simulink model "dvbs2_stream"  (R2024b)
settings: Solver=FixedStepDiscrete  StartTime=0.0  StopTime=18000/Fs  RelTol=1e-3
PreLoadFcn:
  | Rs = 125e3;
  | Fs = 8*Rs;
  | nsamp = 4096;
  | t = (0:nsamp)/Fs;
  | y = randi(2^8-1,1,2048);
  | ly = length(y);
InitFcn:
  | Rs = 125e3;
  | Fs = 8*Rs;
  | nsamp = 4096;
  | t = (0:nsamp)/Fs;
  | y = randi(2^8-1,1,2048);
  | ly = length(y);
libraries: hdlsllib x132, simulink x41, dspsigops x7, commseqgen3 x5, whdlutilities x5, commhdlcrc x2, dsphdlfiltering2 x1, whdlmod x1, sdrzblksprivate x1
(part 2 of 6)

== system dvbs2_stream/HDL_DUT/Tx/DVB-S2 Tx/BB Frame Generator/Multiplexer ==
  dataBits : Inport
  dataValid : Inport  Port=2
  dataEnd : Inport  Port=3
  headerBits : Inport  Port=4
  headerStart : Inport  Port=5
  headerValid : Inport  Port=6
  MODCOD : Inport  Port=7
  FECFrame : Inport  Port=8
  Delay{,1..3} (4 alike) : Delay
  Delay4 : Delay  DelayLength=1
  Delay5 : Delay  DelayLength=1
  Logical Operator : Logic  Operator=OR  AllPortsSameDT=off  OutDataTypeStr=boolean
  No HDL : Subsystem
  Switch : Switch  Criteria=u2 ~= 0  SaturateOnIntegerOverflow=off  InputSameDT=off
  dataOut : Outport
  startOut : Outport  Port=2
  endOut : Outport  Port=3
  validOut : Outport  Port=4
  MODCODOut : Outport  Port=5
  FECFrameOut : Outport  Port=6
  wires:
  FECFrame/1 -> Delay5/1
  Delay5/1 -> FECFrameOut/1
  Delay4/1 -> MODCODOut/1
  Delay3/1 -> endOut/1
  Delay2/1 -> startOut/1
  Delay1/1 -> validOut/1
  Delay/1 -> dataOut/1
  dataValid/1 -> No HDL/1(dvalid), Logical Operator/1, Switch/2
  MODCOD/1 -> Delay4/1
  Logical Operator/1 -> Delay1/1
  Switch/1 -> Delay/1
  headerValid/1 -> No HDL/2(hvalid), Logical Operator/2
  headerBits/1 -> Switch/3
  dataBits/1 -> Switch/1
  dataEnd/1 -> Delay3/1
  headerStart/1 -> Delay2/1

== system dvbs2_stream/HDL_DUT/Tx/DVB-S2 Tx/FEC Encoder/DVB-S2 BCH Encoder ==
  dataIn : Inport
  ctrlIn : Inport  Port=2
  frameType : Inport  Port=3
  codeRateIdx : Inport  Port=4
  Input controller : Subsystem
  Output Controller : Subsystem
  Parity Generation : Subsystem
  Store and Retreive Input : Subsystem
  Terminator : Terminator
  dataOut : Outport
  ctrlOut : Outport  Port=2
  wires:
  Store and Retreive Input/2(outrd_data) -> Parity Generation/1(outrd_data)
  Store and Retreive Input/3(outRd_valid) -> Parity Generation/2(outRd_valid)
  Output Controller/1(outData) -> dataOut/1
  Output Controller/2(outCtrl) -> ctrlOut/1
  Store and Retreive Input/4(ParityCalCompFlag) -> Parity Generation/3(ParityCalCompFlag)
  Parity Generation/3(parityScalarOut) -> Output Controller/4(outputParity)
  Parity Generation/4(parityScalarValidOut) -> Output Controller/5(validParity)
  Output Controller/3(nxtFrame) -> Terminator/1
  Input controller/6(reset) -> Store and Retreive Input/7(resetIn)
  ctrlIn/1 -> Input controller/1(ctrlIn)
  frameType/1 -> Input controller/2(frameType)
  codeRateIdx/1 -> Input controller/3(codeRateIdx)
  Input controller/1(iwr_enb) -> Store and Retreive Input/2(iwr_enb)
  Input controller/8(sampledStartIn) -> Output Controller/8(sampledStartIn)
  Input controller/2(iwr_addr) -> Store and Retreive Input/3(iwr_addr)
  Input controller/5(framLenDelayed) -> Store and Retreive Input/6(framLenDelayed)
  Input controller/3(ird_addr) -> Store and Retreive Input/4(ird_addr)
  Input controller/7(parLen) -> Output Controller/7(parLen), Parity Generation/5(parLen)
  Input controller/4(ird_valid) -> Store and Retreive Input/5(ird_valid)
  Input controller/11(frameLen) -> Output Controller/11(frameLen)
  Input controller/12(validCodeRate) -> Output Controller/12(validCodeRate)
  Input controller/13(unitFrameLen) -> Output Controller/13(unitFrameLen)
  dataIn/1 -> Store and Retreive Input/1(iwr_data)
  Store and Retreive Input/5(resetOut) -> Parity Generation/4(resetIn)
  Parity Generation/5(resetOut) -> Output Controller/6(resetIn)
  Parity Generation/1(readDataOut) -> Output Controller/2(outputMsg)
  Parity Generation/2(readValidOut) -> Output Controller/3(validMsg)
  Store and Retreive Input/1(framLenDelay) -> Output Controller/1(framLenDelayed)
  Input controller/9(enbBCHEnc) -> Output Controller/9(enbBCHEnc)
  Input controller/10(sampledEndIn) -> Output Controller/10(sampledEndIn)

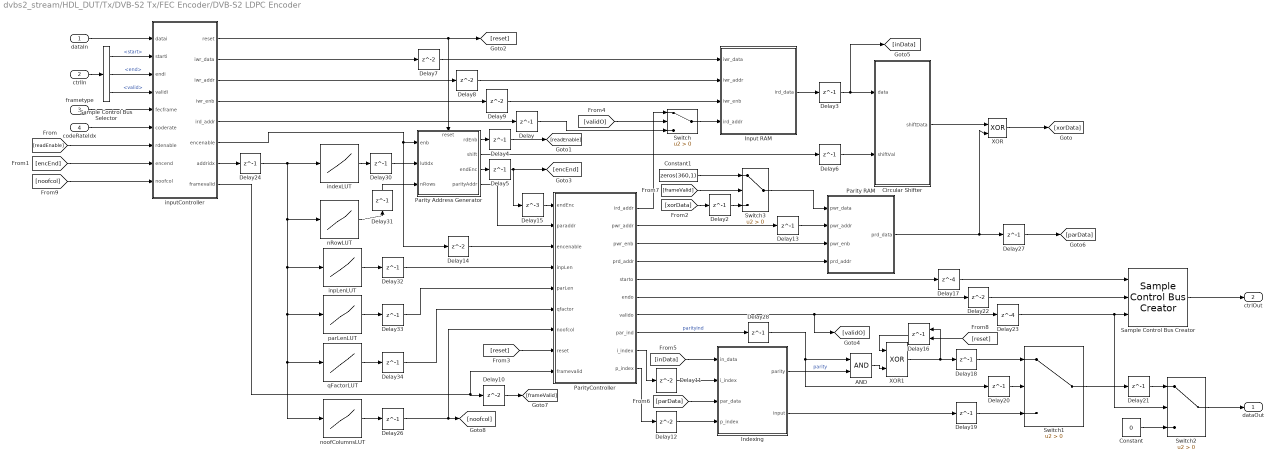
== system dvbs2_stream/HDL_DUT/Tx/DVB-S2 Tx/FEC Encoder/DVB-S2 LDPC Encoder ==
  dataIn : Inport
  ctrlIn : Inport  Port=2
  frametype : Inport  Port=3
  codeRateIdx : Inport  Port=4
  AND : Logic  IconShape=distinctive  AllPortsSameDT=off  OutDataTypeStr=boolean
  Circular Shifter : Subsystem
  Constant : Constant  Value=0  OutDataTypeStr=boolean  SampleTime=-1
  Constant1 : Constant  Value=zeros(360,1)  OutDataTypeStr=boolean  SampleTime=-1
  Delay{,2..6,13,18..21,24,26..28,30..34} (20 alike) : Delay  DelayLength=1
  Delay{7..10,14,22} (6 alike) : Delay
  Delay11 : Delay  InitialCondition=1
  Delay12 : Delay  InitialCondition=1
  Delay15 : Delay  DelayLength=3
  Delay16 : Delay  DelayLength=1  ExternalReset=Level
      settings: InputPortMap=u0,r5
  Delay17 : Delay  DelayLength=4
  Delay23 : Delay  DelayLength=4  InitialCondition=0
  Indexing : MATLAB Function  TreatAsAtomicUnit=on
  Input RAM : Subsystem  TreatAsAtomicUnit=on
  Parity Address Generator : Subsystem
      settings: PortSchema="{\"entries\":[{\"content\":{\"sides\":[{\"content\":{\"connectorIds\":[\"In1\",\"In2\",\"In3\"]},\"type\":\"ConnectorPlacement.EquallySpacedRectSide\",\"uuid\":\"3d7dec72-7252-434a-9e41-e0042beb8f81\"},{\"content\":{\"connectorIds\":[\"Out1\",\"Out2\",\"Out3\",\"Out4\"],\"side\":\"RIGHT\"},\"type\":\"ConnectorPlacement.EquallySpacedRectSide\",\"uuid\":\"b52d290b-db9d-4f8b-b785-ddc131f6f7c7\"},{\"content\":{\"connectorIds\":[\"In4\"],\"side\":\"TOP\"},\"type\":\"ConnectorPlacement.EquallySpacedRectSide\",\"uuid\":\"6c6734b1-a517-4502-8814-67d54e3edf46\"}]},\"type\":\"ConnectorPlacement.EquallySpacedConnector\",\"uuid\":\"7bd65a32-b8b8-4f3b-b937-2885ab80089c\"}],\"packageUris\":[\"http://schema.mathworks.com/mf0/Connector/R2020b\"],\"version\":\"1.0\"}"
  Parity RAM : Subsystem  TreatAsAtomicUnit=on
  ParityController : MATLAB Function  TreatAsAtomicUnit=on
  Sample Control Bus Creator : whdlutilities/Sample Control Bus Creator
  Sample Control Bus Selector : whdlutilities/Sample Control Bus Selector  OutputSignals=start,end,valid
  Switch{,1..3} (4 alike) : Switch  Criteria=u2 > Threshold  SaturateOnIntegerOverflow=off  InputSameDT=off
  XOR : Logic  Operator=XOR  IconShape=distinctive  AllPortsSameDT=off  OutDataTypeStr=boolean
  XOR1 : Logic  Operator=XOR  IconShape=distinctive  AllPortsSameDT=off  OutDataTypeStr=fixdt(0,1,0)
  indexLUT : Lookup_n-D  NumberOfTableDimensions=1  BreakpointsSpecification=Even spacing  BreakpointsForDimension1=[1:20]  BreakpointsForDimension1FirstPoint=0  Table=[0,45,105,177,267,375,495,630,774,924,1084,1246,1246,1246,1246,1246,1246,1255,1270,1288,1308,1335,1365,1398,1433,1470,1510,1510,1510,1510,1510,1510]  InterpMethod=Flat  RemoveProtectionInput=on  InternalRulePriority=Speed  OutDataTypeStr=fixdt(0,11,0)  RndMeth=Simplest
  inpLenLUT : Lookup_n-D  NumberOfTableDimensions=1  BreakpointsSpecification=Even spacing  BreakpointsForDimension1=[1:20]  BreakpointsForDimension1FirstPoint=0  Table=[16200,21600,25920,32400,38880,43200,48600,51840,54000,57600,58320,58320,58320,58320,58320,58320,3240,5400,6480,7200,9720,10800,11880,12600,13320,14400,14400,14400,14400,14400,14400,14400]  InterpMethod=Flat  RemoveProtectionInput=on  InternalRulePriority=Speed  OutDataTypeStr=fixdt(0,16,0)  RndMeth=Simplest
  inputController : MATLAB Function  TreatAsAtomicUnit=on
  nRowLUT : Lookup_n-D  NumberOfTableDimensions=1  BreakpointsSpecification=Even spacing  BreakpointsForDimension1=[1:20]  BreakpointsForDimension1FirstPoint=0  Table=[45,60,72,90,108,120,135,144,150,160,162,162,162,162,162,162,9,15,18,20,27,30,33,35,37,40,40,40,40,40,40,40]  InterpMethod=Flat  RemoveProtectionInput=on  InternalRulePriority=Speed  OutDataTypeStr=fixdt(0,8,0)  RndMeth=Simplest
  noofColumnsLUT : Lookup_n-D  NumberOfTableDimensions=1  BreakpointsSpecification=Even spacing  BreakpointsForDimension1=[1:20]  BreakpointsForDimension1FirstPoint=0  Table=[45,60,72,90,108,120,135,144,150,160,162,162,162,162,162,162,9,15,18,20,27,30,33,35,37,40,40,40,40,40,40,40]  InterpMethod=Flat  RemoveProtectionInput=on  InternalRulePriority=Speed  OutDataTypeStr=uint8  RndMeth=Simplest
  parLenLUT : Lookup_n-D  NumberOfTableDimensions=1  BreakpointsSpecification=Even spacing  BreakpointsForDimension1=[1:20]  BreakpointsForDimension1FirstPoint=0  Table=[48600,43200,38880,32400,25920,21600,16200,12960,10800,7200,6480,6480,6480,6480,6480,6480,12960,10800,9720,9000,6480,5400,4320,3600,2880,1800,1800,1800,1800,1800,1800,1800]  InterpMethod=Flat  RemoveProtectionInput=on  InternalRulePriority=Speed  OutDataTypeStr=fixdt(0,16,0)  RndMeth=Simplest
  qFactorLUT : Lookup_n-D  NumberOfTableDimensions=1  BreakpointsSpecification=Even spacing  BreakpointsForDimension1=[1:20]  BreakpointsForDimension1FirstPoint=0  Table=[135,120,108,90,72,60,45,36,30,20,18,18,18,18,18,18,36,30,27,25,18,15,12,10,8,5,5,5,5,5,5,5]  InterpMethod=Flat  RemoveProtectionInput=on  InternalRulePriority=Speed  OutDataTypeStr=fixdt(0,9,0)  RndMeth=Simplest
  dataOut : Outport
  ctrlOut : Outport  Port=2
  wires:
  ParityController/3(pwr_enb) -> Parity RAM/3(pwr_enb)
  noofColumnsLUT/1 -> Delay26/1
  [frameValid] -> Switch3/2
  Input RAM/1(ird_data) -> Delay3/1
  inputController/2(iwr_data) -> Delay7/1
  [xorData] -> Delay2/1
  Delay10/1 -> [frameValid]
  Constant/1 -> Switch2/3
  [noofcol] -> inputController/9(noofcol)
  inputController/6(encenable) -> Parity Address Generator/1(enb), Delay14/1
  [encEnd] -> inputController/8(encend)
  Indexing/2(input) -> Delay19/1
  Delay23/1 -> Switch2/2, Sample Control Bus Creator/3
  ParityController/4(prd_addr) -> Parity RAM/4(prd_addr)
  [reset] -> ParityController/8(reset)
  Delay17/1 -> Sample Control Bus Creator/1
  Delay21/1 -> Switch2/1
  [parData] -> Indexing/3(par_data)
  Delay26/1 -> [noofcol], ParityController/7(noofcol)
  Switch1/1 -> Delay21/1
  Delay33/1 -> ParityController/5(parLen)
  Delay7/1 -> Input RAM/1(iwr_data)
  frametype/1 -> inputController/5(fecframe)
  Delay32/1 -> ParityController/4(inpLen)
  ParityController/1(ird_addr) -> Switch/1
  Delay24/1 -> indexLUT/1, nRowLUT/1, inpLenLUT/1, parLenLUT/1, qFactorLUT/1, noofColumnsLUT/1
  ParityController/6(endo) -> Delay22/1
  Parity Address Generator/1(rdEnb) -> Delay4/1
  Delay11/1 -> Indexing/2(i_index)
  nRowLUT/1 -> Delay31/1
  inputController/5(ird_addr) -> Delay/1
  Sample Control Bus Selector/2 -> inputController/3(endi)  "<end>"
  ParityController/2(pwr_addr) -> Delay13/1
  Delay9/1 -> Input RAM/3(iwr_enb)
  Delay14/1 -> ParityController/3(encenable)
  inpLenLUT/1 -> Delay32/1
  ParityController/10(p_index) -> Delay12/1
  Delay19/1 -> Switch1/3
  [readEnable] -> inputController/7(rdenable)
  Parity Address Generator/3(endEnc) -> Delay5/1
  Delay30/1 -> Parity Address Generator/2(lutIdx)
  Parity Address Generator/4(parityAddr) -> ParityController/2(paraddr)
  [validO] -> Switch/2
  indexLUT/1 -> Delay30/1
  [inData] -> Indexing/1(in_data)
  Sample Control Bus Selector/1 -> inputController/2(starti)  "<start>"
  Delay28/1 -> AND/1, Delay20/1
  Indexing/1(parity) -> AND/2  "parity"
  Delay3/1 -> Circular Shifter/1(data), [inData]
  ctrlIn/1 -> Sample Control Bus Selector/1
  ParityController/8(par_ind) -> Delay28/1  "parityInd"
  Sample Control Bus Creator/1 -> ctrlOut/1
  Delay31/1 -> Parity Address Generator/3(nRows)
  inputController/1(reset) -> [reset], Parity Address Generator/4(reset)
  Delay16/1 -> XOR1/1
  Delay13/1 -> Parity RAM/2(pwr_addr)
  Switch2/1 -> dataOut/1
  AND/1 -> XOR1/2
  Delay12/1 -> Indexing/4(p_index)
  qFactorLUT/1 -> Delay34/1
  ParityController/5(starto) -> Delay17/1
  Delay/1 -> Switch/3
  Delay22/1 -> Sample Control Bus Creator/2
  XOR1/1 -> Delay18/1, Delay16/1
  Delay5/1 -> Delay15/1, [encEnd]
  Parity RAM/1(prd_data) -> XOR/2, Delay27/1
  ParityController/9(i_index) -> Delay11/1
  codeRateIdx/1 -> inputController/6(coderate)
  Switch3/1 -> Parity RAM/1(pwr_data)
  Delay27/1 -> [parData]
  Delay4/1 -> [readEnable]
  Switch/1 -> Input RAM/4(ird_addr)
  Circular Shifter/1(shiftData) -> XOR/1
  Constant1/1 -> Switch3/1
  dataIn/1 -> inputController/1(datai)
  Delay15/1 -> ParityController/1(endEnc)
  Delay34/1 -> ParityController/6(qfactor)
  Delay2/1 -> Switch3/3
  Delay8/1 -> Input RAM/2(iwr_addr)
  Delay6/1 -> Circular Shifter/2(shiftVal)
  parLenLUT/1 -> Delay33/1
  Delay20/1 -> Switch1/2
  inputController/3(iwr_addr) -> Delay8/1
  inputController/8(framevalid) -> ParityController/9(framevalid), Delay10/1
  Sample Control Bus Selector/3 -> inputController/4(validi)  "<valid>"
  inputController/4(iwr_enb) -> Delay9/1
  inputController/7(addridx) -> Delay24/1
  Delay18/1 -> Switch1/1
  XOR/1 -> [xorData]
  ParityController/7(valido) -> Delay23/1, [validO]
  Parity Address Generator/2(shift) -> Delay6/1
  [reset] -> Delay16/2

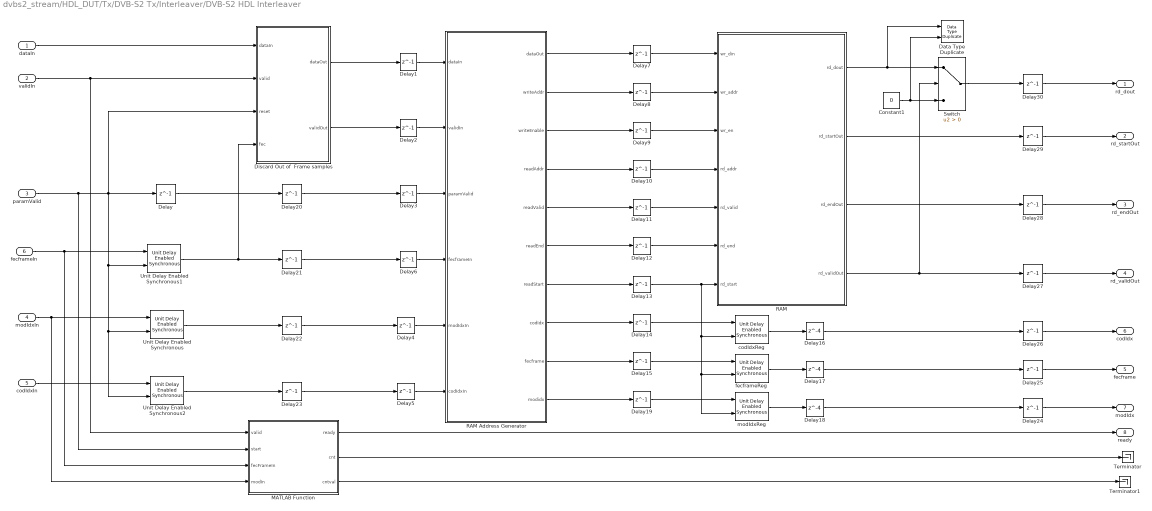
== system dvbs2_stream/HDL_DUT/Tx/DVB-S2 Tx/Interleaver/DVB-S2 HDL Interleaver ==
  dataIn : Inport
  validIn : Inport  Port=2
  paramValid : Inport  Port=3
  modIdxIn : Inport  Port=4
  codIdxIn : Inport  Port=5
  fecframeIn : Inport  Port=6
  Constant1 : Constant  Value=0  OutDataTypeStr=Inherit: Inherit via back propagation  SampleTime=Tsamp
  Data Type Duplicate : DataTypeDuplicate
  Delay{,1..15,19..30} (28 alike) : Delay  DelayLength=1
  Delay16 : Delay  DelayLength=4
  Delay17 : Delay  DelayLength=4
  Delay18 : Delay  DelayLength=4
  Discard Out of  Frame samples : MATLAB Function  TreatAsAtomicUnit=on
  MATLAB Function : MATLAB Function  TreatAsAtomicUnit=on
  RAM : Subsystem
  RAM Address Generator : Subsystem
  Switch : Switch  Criteria=u2 > Threshold  SaturateOnIntegerOverflow=off  InputSameDT=off
  Terminator : Terminator
  Terminator1 : Terminator
  Unit Delay Enabled Synchronous : hdlsllib/Discrete/Unit Delay Enabled Synchronous  InitialCondition=0.0  SampleTime=-1
  Unit Delay Enabled Synchronous1 : hdlsllib/Discrete/Unit Delay Enabled Synchronous  InitialCondition=0.0  SampleTime=-1
  Unit Delay Enabled Synchronous2 : hdlsllib/Discrete/Unit Delay Enabled Synchronous  InitialCondition=0.0  SampleTime=-1
  codIdxReg : hdlsllib/Discrete/Unit Delay Enabled Synchronous  InitialCondition=0.0  SampleTime=-1
  fecframeReg : hdlsllib/Discrete/Unit Delay Enabled Synchronous  InitialCondition=0.0  SampleTime=-1
  modIdxReg : hdlsllib/Discrete/Unit Delay Enabled Synchronous  InitialCondition=0.0  SampleTime=-1
  rd_dout : Outport
  rd_startOut : Outport  Port=2
  rd_endOut : Outport  Port=3
  rd_validOut : Outport  Port=4
  fecframe : Outport  Port=5
  codIdx : Outport  Port=6
  modIdx : Outport  Port=7
  ready : Outport  Port=8
  wires:
  Delay30/1 -> rd_dout/1
  Delay29/1 -> rd_startOut/1
  Delay28/1 -> rd_endOut/1
  Delay27/1 -> rd_validOut/1
  Delay26/1 -> codIdx/1
  Delay25/1 -> fecframe/1
  Delay24/1 -> modIdx/1
  MATLAB Function/3(cntval) -> Terminator1/1
  MATLAB Function/2(cnt) -> Terminator/1
  MATLAB Function/1(ready) -> ready/1
  RAM/2(rd_startOut) -> Delay29/1
  Delay23/1 -> Delay5/1
  Delay22/1 -> Delay4/1
  Delay21/1 -> Delay6/1
  Delay20/1 -> Delay3/1
  Discard Out of  Frame samples/1(dataOut) -> Delay1/1
  Constant1/1 -> Switch/3, Data Type Duplicate/2
  Switch/1 -> Delay30/1
  Discard Out of  Frame samples/2(validOut) -> Delay2/1
  Unit Delay Enabled Synchronous/1 -> Delay22/1
  Unit Delay Enabled Synchronous2/1 -> Delay23/1
  Unit Delay Enabled Synchronous1/1 -> Delay21/1, Discard Out of  Frame samples/4(fec)
  Delay/1 -> Delay20/1
  Delay19/1 -> modIdxReg/1
  RAM Address Generator/10(modidx) -> Delay19/1
  Delay18/1 -> Delay24/1
  modIdxReg/1 -> Delay18/1
  RAM Address Generator/5(readValid) -> Delay11/1
  RAM Address Generator/8(codIdx) -> Delay14/1
  RAM Address Generator/2(writeAddr) -> Delay8/1
  RAM Address Generator/4(readAddr) -> Delay10/1
  RAM Address Generator/7(readStart) -> Delay13/1
  RAM Address Generator/6(readEnd) -> Delay12/1
  RAM Address Generator/9(fecframe) -> Delay15/1
  RAM Address Generator/3(writeEnable) -> Delay9/1
  dataIn/1 -> Discard Out of  Frame samples/1(dataIn)
  RAM Address Generator/1(dataOut) -> Delay7/1
  validIn/1 -> Discard Out of  Frame samples/2(valid), MATLAB Function/1(valid)
  RAM/4(rd_validOut) -> Delay27/1, Switch/2
  paramValid/1 -> MATLAB Function/2(start), Unit Delay Enabled Synchronous1/2, Unit Delay Enabled Synchronous/2, Unit Delay Enabled Synchronous2/2, Delay/1, Discard Out of  Frame samples/3(reset)
  codIdxIn/1 -> Unit Delay Enabled Synchronous2/1
  modIdxIn/1 -> MATLAB Function/4(modIn), Unit Delay Enabled Synchronous/1
  fecframeIn/1 -> MATLAB Function/3(fecFrameIn), Unit Delay Enabled Synchronous1/1
  RAM/3(rd_endOut) -> Delay28/1
  fecframeReg/1 -> Delay17/1
  RAM/1(rd_dout) -> Switch/1, Data Type Duplicate/1
  codIdxReg/1 -> Delay16/1
  Delay1/1 -> RAM Address Generator/1(dataIn)
  Delay2/1 -> RAM Address Generator/2(validIn)
  Delay3/1 -> RAM Address Generator/3(paramValid)
  Delay4/1 -> RAM Address Generator/5(modIdxIn)
  Delay5/1 -> RAM Address Generator/6(codIdxIn)
  Delay6/1 -> RAM Address Generator/4(fecframeIn)
  Delay7/1 -> RAM/1(wr_din)
  Delay8/1 -> RAM/2(wr_addr)
  Delay9/1 -> RAM/3(wr_en)
  Delay10/1 -> RAM/4(rd_addr)
  Delay11/1 -> RAM/5(rd_valid)
  Delay12/1 -> RAM/6(rd_end)
  Delay13/1 -> RAM/7(rd_start), fecframeReg/2, modIdxReg/2, codIdxReg/2
  Delay14/1 -> codIdxReg/1
  Delay15/1 -> fecframeReg/1
  Delay16/1 -> Delay26/1
  Delay17/1 -> Delay25/1

== system dvbs2_stream/HDL_DUT/Tx/DVB-S2 Tx/No HDL/Subsystem ==
  In1 : Inport
  Enable : EnablePort
  To Workspace : ToWorkspace  VariableName=simDummyFrameNos  SaveFormat=Timeseries  SampleTime=-1
      settings: Save2DSignal=2-D array (concatenate along first dimension)
  wires:
  In1/1 -> To Workspace/1

== system dvbs2_stream/HDL_DUT/Tx/DVB-S2 Tx/PL Frame Generator/Frame Length ==
  fecframe : Inport
  modIdx : Inport  Port=2
  Delay2 : Delay  DelayLength=1
  Delay3 : Delay  DelayLength=8
  Normal Frame xFECFrame Length : Lookup_n-D  NumberOfTableDimensions=1  BreakpointsSpecification=Even spacing  BreakpointsForDimension1=[-5:5]  BreakpointsForDimension1FirstPoint=0  Table=64800./log2([4 8 16 32])  TableDataTypeStr=fixdt(0,15,0)  InterpMethod=Flat  InternalRulePriority=Speed  OutDataTypeStr=fixdt(0,15,0)  RndMeth=Simplest
  Short Frame xFECFrame Length : Lookup_n-D  NumberOfTableDimensions=1  BreakpointsSpecification=Even spacing  BreakpointsForDimension1=[-5:5]  BreakpointsForDimension1FirstPoint=0  Table=16200./log2([4 8 16 32])  TableDataTypeStr=fixdt(0,15,0)  InterpMethod=Flat  InternalRulePriority=Speed  OutDataTypeStr=fixdt(0,15,0)  RndMeth=Simplest
  Switch : Switch  Criteria=u2 ~= 0  SaturateOnIntegerOverflow=off  InputSameDT=off
  xFECFrameLength : Outport
  wires:
  Delay3/1 -> Delay2/1
  Delay2/1 -> xFECFrameLength/1
  modIdx/1 -> Normal Frame xFECFrame Length/1, Short Frame xFECFrame Length/1
  fecframe/1 -> Switch/2
  Normal Frame xFECFrame Length/1 -> Switch/3
  Short Frame xFECFrame Length/1 -> Switch/1
  Switch/1 -> Delay3/1

== system dvbs2_stream/HDL_DUT/Tx/DVB-S2 Tx/PL Frame Generator/Multiplexer ==
  plheaderData : Inport
  plheaderStart : Inport  Port=2
  plheaderEnd : Inport  Port=3
  plheaderValid : Inport  Port=4
  pilotdata : Inport  Port=5
  pilotEnd : Inport  Port=6
  pilotValid : Inport  Port=7
  slotsData : Inport  Port=8
  data16SlotsEnd : Inport  Port=9
  slotsValid : Inport  Port=10
  dummyData : Inport  Port=11
  dummyValid : Inport  Port=12
  dummyHeaderSrt : Inport  Port=13
  dummyHeaderEnd : Inport  Port=14
  Logical Operator : Logic  Operator=OR  AllPortsSameDT=off  OutDataTypeStr=boolean
  Logical Operator2 : Logic  Operator=OR  Inputs=4  AllPortsSameDT=off  OutDataTypeStr=boolean
  Logical Operator3 : Logic  Operator=OR  AllPortsSameDT=off  OutDataTypeStr=boolean
  Multiport Switch : MultiPortSwitch  DataPortOrder=Zero-based contiguous  Inputs=4  zeroidx=on  SaturateOnIntegerOverflow=off  InputSameDT=off
  No HDL : Subsystem
  Priority Encoder : MATLAB Function  TreatAsAtomicUnit=on
  Terminator : Terminator
  Terminator11 : Terminator
  dataOut : Outport
  startOfPlheader : Outport  Port=2
  endOfPlheader : Outport  Port=3
  validOut : Outport  Port=4
  wires:
  Logical Operator3/1 -> endOfPlheader/1
  Logical Operator/1 -> startOfPlheader/1
  dummyHeaderEnd/1 -> Logical Operator3/1
  dummyHeaderSrt/1 -> Logical Operator/1
  dummyData/1 -> Multiport Switch/5
  slotsData/1 -> Multiport Switch/4
  pilotdata/1 -> Multiport Switch/3
  plheaderData/1 -> Multiport Switch/2
  plheaderEnd/1 -> Logical Operator3/2
  Multiport Switch/1 -> dataOut/1
  Priority Encoder/1(y) -> Multiport Switch/1
  dummyValid/1 -> Priority Encoder/4(x4), Logical Operator2/4, No HDL/4(dummyValid)
  plheaderStart/1 -> Logical Operator/2
  Logical Operator2/1 -> validOut/1
  pilotEnd/1 -> Terminator11/1
  plheaderValid/1 -> No HDL/2(In2), Logical Operator2/2, Priority Encoder/1(x1)
  data16SlotsEnd/1 -> Terminator/1
  pilotValid/1 -> No HDL/1(In1), Logical Operator2/1, Priority Encoder/2(x2)
  slotsValid/1 -> Logical Operator2/3, No HDL/3(In5), Priority Encoder/3(x3)

== system dvbs2_stream/HDL_DUT/Tx/DVB-S2 Tx/PL Frame Generator/PL Data Scrambler ==
  dataIn : Inport
  startOfPlheader : Inport  Port=2
  endOfPlheader : Inport  Port=3
  validIn : Inport  Port=4
  Delay1 : Delay  DelayLength=7
  Delay{2..8,10..12,22..26} (15 alike) : Delay  DelayLength=1
  Delay{13..21} (9 alike) : Delay
  Delay9 : Delay  DelayLength=7
  PL Scramble Sequence Mapper LUT : Lookup_n-D  NumberOfTableDimensions=1  LookupTableObject=''  BreakpointsSpecification=Even spacing  BreakpointsForDimension1=[-5:5]  BreakpointsForDimension1FirstPoint=0  BreakpointsForDimension2FirstPoint=10  BreakpointsForDimension2Spacing=12  IndexSearchMethod=Evenly spaced points  Table=[1;1i;-1;-1i]  TableDataTypeStr=fixdt(1,2,0)  InterpMethod=Flat  DiagnosticForOutOfRangeInput=Error  InternalRulePriority=Speed  OutDataTypeStr=fixdt(1,2,0)  RndMeth=Simplest
  PL Scrambler Gold Sequence Generator : Subsystem  mask{n=0}
      mask prompts: n "Index of Gold Sequence :"
  Product : Product  OutDataTypeStr=Inherit: Same as first input
  Switch : Switch  Criteria=u2 ~= 0  SaturateOnIntegerOverflow=off  InputSameDT=off
  Unit Delay Enabled Resettable Synchronous : hdlsllib/Discrete/Unit Delay Enabled Resettable Synchronous  InitialCondition=0.0  SampleTime=-1
  dataOut : Outport
  validOut : Outport  Port=2
  wires:
  Unit Delay Enabled Resettable Synchronous/1 -> Delay1/1
  Delay26/1 -> PL Scrambler Gold Sequence Generator/1(reset), Unit Delay Enabled Resettable Synchronous/3
  Delay25/1 -> PL Scrambler Gold Sequence Generator/2(validIn)
  Delay24/1 -> Delay9/1
  startOfPlheader/1 -> Unit Delay Enabled Resettable Synchronous/1, Unit Delay Enabled Resettable Synchronous/2
  PL Scrambler Gold Sequence Generator/1(dataOut) -> Delay2/1
  Delay11/1 -> Delay14/1
  Delay7/1 -> Delay16/1
  dataIn/1 -> Delay24/1
  PL Scramble Sequence Mapper LUT/1 -> Delay7/1
  Product/1 -> Delay20/1
  Switch/1 -> Delay22/1
  PL Scrambler Gold Sequence Generator/2(validOut) -> Delay5/1
  endOfPlheader/1 -> Delay26/1
  validIn/1 -> Delay25/1
  Delay9/1 -> Delay4/1, Delay6/1
  Delay1/1 -> Delay3/1
  Delay2/1 -> PL Scramble Sequence Mapper LUT/1
  Delay3/1 -> Delay11/1
  Delay4/1 -> Delay10/1
  Delay5/1 -> Delay8/1
  Delay6/1 -> Delay12/1
  Delay8/1 -> Delay17/1
  Delay10/1 -> Delay15/1
  Delay13/1 -> Delay18/1
  Delay14/1 -> Delay19/1
  Delay15/1 -> Product/1
  Delay16/1 -> Product/2
  Delay17/1 -> Delay21/1
  Delay18/1 -> Switch/1
  Delay19/1 -> Switch/2
  Delay20/1 -> Switch/3
  Delay21/1 -> Delay23/1
  Delay22/1 -> dataOut/1
  Delay23/1 -> validOut/1
  Delay12/1 -> Delay13/1

== system dvbs2_stream/HDL_DUT/Tx/DVB-S2 Tx/PL Frame Generator/PL Header Generator ==
  trigger : Inport
  pilotActive : Inport  Port=2
  modcod : Inport  Port=3
  fecframe : Inport  Port=4
  Delay{,1..3} (4 alike) : Delay  DelayLength=1
  PL Header Bits Generator : Subsystem
  Terminator : Terminator
  Terminator1 : Terminator
  piby2 BPSK Modulator : Subsystem
  dataOut : Outport
  validOut : Outport  Port=2
  wires:
  piby2 BPSK Modulator/2(startOut) -> Terminator/1
  piby2 BPSK Modulator/1(dataOut) -> dataOut/1
  piby2 BPSK Modulator/3(endOut) -> Terminator1/1
  PL Header Bits Generator/3(bitsEnd) -> piby2 BPSK Modulator/3(endIn)
  PL Header Bits Generator/2(bitsStart) -> piby2 BPSK Modulator/2(startIn)
  piby2 BPSK Modulator/4(validOut) -> validOut/1
  PL Header Bits Generator/4(bitsValid) -> piby2 BPSK Modulator/4(validIn)
  PL Header Bits Generator/1(bitsOut) -> piby2 BPSK Modulator/1(bitsIn)
  Delay3/1 -> PL Header Bits Generator/1(trigger)
  Delay2/1 -> PL Header Bits Generator/2(pilotActive)
  Delay1/1 -> PL Header Bits Generator/3(modcod)
  Delay/1 -> PL Header Bits Generator/4(fecframe)
  pilotActive/1 -> Delay2/1
  modcod/1 -> Delay1/1
  fecframe/1 -> Delay/1
  trigger/1 -> Delay3/1

== system dvbs2_stream/HDL_DUT/Tx/DVB-S2 Tx/PL Frame Generator/RAM FIFO ==
  dataIn : Inport
  validIn : Inport  Port=2
  dataIn1 : Inport  Port=3
  startIn1 : Inport  Port=4
  validIn1 : Inport  Port=5
  frameLength : Inport  Port=6
  PL Data FIFO : Subsystem
      settings: PortSchema="{\"entries\":[{\"content\":{\"sides\":[{\"content\":{\"connectorIds\":[\"In1\",\"In2\",\"Out8\",\"In3\",\"In4\",\"In5\",\"In6\"]},\"type\":\"ConnectorPlacement.EquallySpacedRectSide\",\"uuid\":\"8624b1c3-ba7c-4e35-b094-1d3a75bbb5aa\"},{\"content\":{\"connectorIds\":[\"Out1\",\"Out2\",\"Out3\",\"Out4\",\"Out5\",\"Out6\",\"Out7\"],\"side\":\"RIGHT\"},\"type\":\"ConnectorPlacement.EquallySpacedRectSide\",\"uuid\":\"28b8a943-c986-4665-8db5-1a3b0585df3a\"},{\"content\":{\"connectorIds\":[],\"side\":\"TOP\"},\"type\":\"ConnectorPlacement.EquallySpacedRectSide\",\"uuid\":\"814d6e08-8c72-454b-9b48-c3c62ce2dfb2\"}]},\"type\":\"ConnectorPlacement.EquallySpacedConnector\",\"uuid\":\"82423169-df73-4f70-a83d-ba96081f6481\"}],\"packageUris\":[\"http://schema.mathworks.com/mf0/Connector/R2020b\"],\"version\":\"1.0\"}"
  PL Header FIFO : Subsystem
      settings: PortSchema="{\"entries\":[{\"content\":{\"sides\":[{\"content\":{\"connectorIds\":[\"In1\",\"In2\",\"In3\",\"Out5\"]},\"type\":\"ConnectorPlacement.EquallySpacedRectSide\",\"uuid\":\"17ee1903-61f4-462b-918b-37a4577cd6d5\"},{\"content\":{\"connectorIds\":[\"Out1\",\"Out2\",\"Out3\",\"Out4\"],\"side\":\"RIGHT\"},\"type\":\"ConnectorPlacement.EquallySpacedRectSide\",\"uuid\":\"53e99393-0da1-48e4-bd02-4cd54a66bf15\"},{\"content\":{\"connectorIds\":[],\"side\":\"TOP\"},\"type\":\"ConnectorPlacement.EquallySpacedRectSide\",\"uuid\":\"3f5b7744-cb83-4728-90ec-96c952f929fa\"}]},\"type\":\"ConnectorPlacement.EquallySpacedConnector\",\"uuid\":\"7c0ee041-1408-4d92-8895-be25a9dc4cb3\"}],\"packageUris\":[\"http://schema.mathworks.com/mf0/Connector/R2020b\"],\"version\":\"1.0\"}"
  Pilot Generator : Subsystem
      settings: PortSchema="{\"entries\":[{\"content\":{\"sides\":[{\"content\":{\"connectorIds\":[\"Out4\"]},\"type\":\"ConnectorPlacement.EquallySpacedRectSide\",\"uuid\":\"60393444-e96f-4a49-aa63-e73913838962\"},{\"content\":{\"connectorIds\":[\"Out1\",\"Out2\",\"Out3\",\"In1\"],\"side\":\"RIGHT\"},\"type\":\"ConnectorPlacement.EquallySpacedRectSide\",\"uuid\":\"bbfeed4a-cbdf-4f6b-9c28-37958929d3d3\"},{\"content\":{\"connectorIds\":[],\"side\":\"TOP\"},\"type\":\"ConnectorPlacement.EquallySpacedRectSide\",\"uuid\":\"3a1e215d-56d0-454b-a618-c727de9dda1a\"}]},\"type\":\"ConnectorPlacement.EquallySpacedConnector\",\"uuid\":\"0bef8ac2-da74-4396-b0bf-efe44cab5a13\"}],\"packageUris\":[\"http://schema.mathworks.com/mf0/Connector/R2020b\"],\"version\":\"1.0\"}"
  plheaderData : Outport
  plheaderStart : Outport  Port=2
  plheaderEnd : Outport  Port=3
  plheaderValid : Outport  Port=4
  pilotData : Outport  Port=5
  pilotEnd : Outport  Port=6
  pilotValid : Outport  Port=7
  slotsData : Outport  Port=8
  data16SlotsEnd : Outport  Port=9
  slotsValid : Outport  Port=10
  dummyData : Outport  Port=11
  dummyValid : Outport  Port=12
  dummyHeaderSrt : Outport  Port=13
  dummyHeaderEnd : Outport  Port=14
  wires:
  PL Data FIFO/7(dummyHeaderEnd) -> dummyHeaderEnd/1
  PL Data FIFO/6(dummyHeaderSrt) -> dummyHeaderSrt/1
  PL Data FIFO/5(dummyValid) -> dummyValid/1
  PL Data FIFO/4(dummyData) -> dummyData/1
  startIn1/1 -> PL Data FIFO/4(startIn)
  PL Header FIFO/5(endOut1) -> PL Data FIFO/2(endOfPLHeader)
  Pilot Generator/3(validOut) -> pilotValid/1
  PL Header FIFO/2(startOut) -> plheaderStart/1
  PL Data FIFO/2(dataOut) -> slotsData/1
  Pilot Generator/1(dataOut) -> pilotData/1
  frameLength/1 -> PL Data FIFO/6(frameLength)
  validIn1/1 -> PL Data FIFO/5(validIn)
  PL Data FIFO/3(validOut) -> slotsValid/1
  dataIn1/1 -> PL Data FIFO/3(dataIn)
  PL Header FIFO/1(dataOut) -> plheaderData/1
  validIn/1 -> PL Header FIFO/2(validIn)
  Pilot Generator/2(endOut) -> pilotEnd/1
  PL Header FIFO/3(endOut) -> plheaderEnd/1
  PL Header FIFO/4(validOut) -> plheaderValid/1
  dataIn/1 -> PL Header FIFO/1(dataIn)
  PL Data FIFO/1(endOf16Slots) -> Pilot Generator/1(trigger), data16SlotsEnd/1
  Pilot Generator/4(endOut1) -> PL Data FIFO/1(endOfPilotBlk)
  PL Data FIFO/8(nextFrameReady) -> PL Header FIFO/3(nextFrameReady)

== system dvbs2_stream/HDL_DUT/Tx/DVB-S2 Tx/PL Frame Generator/Subsystem ==
  data : Inport
  start : Inport  Port=2
  endIn : Inport  Port=3
  validIn : Inport  Port=4
  8x : MATLAB Function  TreatAsAtomicUnit=on
  Delay : Delay  DelayLength=8
  Delay1 : Delay  DelayLength=8
  Delay2 : Delay  DelayLength=1
  Unit Delay Enabled Synchronous : hdlsllib/Discrete/Unit Delay Enabled Synchronous  InitialCondition=0.0  SampleTime=-1
  dataOut : Outport
  startOut : Outport  Port=2
  validOut : Outport  Port=3
  wires:
  Delay2/1 -> dataOut/1
  Unit Delay Enabled Synchronous/1 -> Delay2/1
  Delay1/1 -> 8x/2(endIn)
  Delay/1 -> 8x/1(startIn)
  endIn/1 -> Delay1/1
  start/1 -> Delay/1
  validIn/1 -> Unit Delay Enabled Synchronous/2
  data/1 -> Unit Delay Enabled Synchronous/1
  8x/1(startOut) -> startOut/1
  8x/2(validOut) -> validOut/1

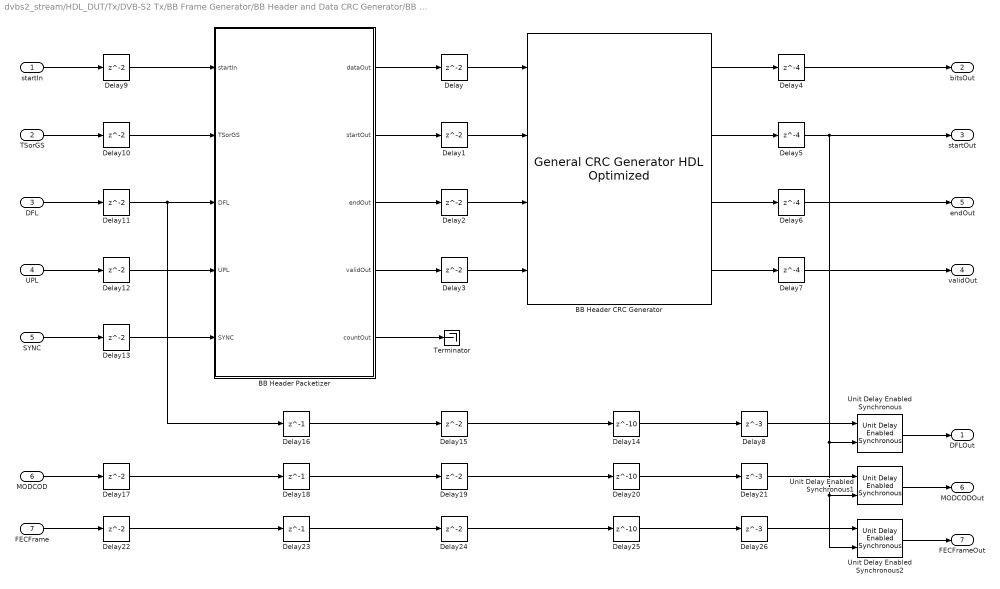
== system dvbs2_stream/HDL_DUT/Tx/DVB-S2 Tx/BB Frame Generator/BB Header and Data CRC Generator/BB Header Generator ==
  startIn : Inport
  TSorGS : Inport  Port=2
  DFL : Inport  Port=3
  UPL : Inport  Port=4
  SYNC : Inport  Port=5
  MODCOD : Inport  Port=6
  FECFrame : Inport  Port=7
  BB Header CRC Generator : commhdlcrc/General CRC Generator HDL Optimized  Polynomial=[1 1 1 0 1 0 1 0 1]  InitialState=0  DirectMethod=off  ReflectInput=off  ReflectCRCChecksum=off  FinalXORValue=0  SimulateUsing=Code generation
  BB Header Packetizer : MATLAB Function  TreatAsAtomicUnit=on
  Delay{,1..3,9..13,15,17,19,22,24} (14 alike) : Delay
  Delay14 : Delay  DelayLength=10
  Delay16 : Delay  DelayLength=1
  Delay18 : Delay  DelayLength=1
  Delay20 : Delay  DelayLength=10
  Delay21 : Delay  DelayLength=3
  Delay23 : Delay  DelayLength=1
  Delay25 : Delay  DelayLength=10
  Delay26 : Delay  DelayLength=3
  Delay{4..7} (4 alike) : Delay  DelayLength=4
  Delay8 : Delay  DelayLength=3
  Terminator : Terminator
  Unit Delay Enabled Synchronous : hdlsllib/Discrete/Unit Delay Enabled Synchronous  InitialCondition=0.0  SampleTime=-1
  Unit Delay Enabled Synchronous1 : hdlsllib/Discrete/Unit Delay Enabled Synchronous  InitialCondition=0.0  SampleTime=-1
  Unit Delay Enabled Synchronous2 : hdlsllib/Discrete/Unit Delay Enabled Synchronous  InitialCondition=0.0  SampleTime=-1
  DFLOut : Outport
  bitsOut : Outport  Port=2
  startOut : Outport  Port=3
  validOut : Outport  Port=4
  endOut : Outport  Port=5
  MODCODOut : Outport  Port=6
  FECFrameOut : Outport  Port=7
  wires:
  Delay26/1 -> Unit Delay Enabled Synchronous2/1
  Delay25/1 -> Delay26/1
  Delay24/1 -> Delay25/1
  Delay23/1 -> Delay24/1
  Delay22/1 -> Delay23/1
  Unit Delay Enabled Synchronous2/1 -> FECFrameOut/1
  FECFrame/1 -> Delay22/1
  Unit Delay Enabled Synchronous1/1 -> MODCODOut/1
  Delay21/1 -> Unit Delay Enabled Synchronous1/1
  Delay20/1 -> Delay21/1
  Delay19/1 -> Delay20/1
  Delay18/1 -> Delay19/1
  Delay17/1 -> Delay18/1
  MODCOD/1 -> Delay17/1
  Delay5/1 -> Unit Delay Enabled Synchronous/2, Unit Delay Enabled Synchronous1/2, Unit Delay Enabled Synchronous2/2, startOut/1
  Unit Delay Enabled Synchronous/1 -> DFLOut/1
  Delay16/1 -> Delay15/1
  Delay11/1 -> Delay16/1, BB Header Packetizer/3(DFL)
  Delay15/1 -> Delay14/1
  Delay14/1 -> Delay8/1
  Delay8/1 -> Unit Delay Enabled Synchronous/1
  Delay13/1 -> BB Header Packetizer/5(SYNC)
  Delay12/1 -> BB Header Packetizer/4(UPL)
  Delay10/1 -> BB Header Packetizer/2(TSorGS)
  Delay9/1 -> BB Header Packetizer/1(startIn)
  Delay7/1 -> validOut/1
  Delay6/1 -> endOut/1
  Delay4/1 -> bitsOut/1
  Delay3/1 -> BB Header CRC Generator/4
  Delay2/1 -> BB Header CRC Generator/3
  Delay1/1 -> BB Header CRC Generator/2
  Delay/1 -> BB Header CRC Generator/1
  BB Header Packetizer/5(countOut) -> Terminator/1
  BB Header CRC Generator/3 -> Delay6/1
  BB Header CRC Generator/4 -> Delay7/1
  BB Header CRC Generator/2 -> Delay5/1
  UPL/1 -> Delay12/1
  BB Header CRC Generator/1 -> Delay4/1
  BB Header Packetizer/1(dataOut) -> Delay/1
  startIn/1 -> Delay9/1
  DFL/1 -> Delay11/1
  BB Header Packetizer/4(validOut) -> Delay3/1
  BB Header Packetizer/2(startOut) -> Delay1/1
  BB Header Packetizer/3(endOut) -> Delay2/1
  SYNC/1 -> Delay13/1
  TSorGS/1 -> Delay10/1

== system dvbs2_stream/HDL_DUT/Tx/DVB-S2 Tx/BB Frame Generator/BB Header and Data CRC Generator/Data Field Generator ==
  dataIn : Inport
  startIn : Inport  Port=2
  endIn : Inport  Port=3
  validIn : Inport  Port=4
  frameEnd : Inport  Port=5
  frameStart : Inport  Port=6
  UPL : Inport  Port=7
  Compare To Constant : simulink/Logic and Bit Operations/Compare To Constant  relop=~=  const=0  OutDataTypeStr=boolean
  Continuous Streams : Subsystem
  Packetized Streams : Subsystem
  Switch{,1..3} (4 alike) : Switch  Criteria=u2 ~= 0  SaturateOnIntegerOverflow=off  InputSameDT=off
  pktBits : Outport
  pktValid : Outport  Port=2
  frameStartOut : Outport  Port=3
  frameEndOut : Outport  Port=4
  wires:
  Compare To Constant/1 -> Switch/2, Switch1/2, Switch2/2, Switch3/2
  UPL/1 -> Compare To Constant/1
  frameStart/1 -> Packetized Streams/6(frameStart), Continuous Streams/4(frameStart)
  frameEnd/1 -> Packetized Streams/5(frameEnd), Continuous Streams/3(frameEnd)
  Continuous Streams/1(dataOut) -> Switch/3
  Continuous Streams/2(validOut) -> Switch1/3
  Continuous Streams/4(frameStartOut) -> Switch3/3
  Continuous Streams/3(frameEndOut) -> Switch2/3
  Switch3/1 -> frameStartOut/1
  Switch2/1 -> frameEndOut/1
  Switch1/1 -> pktValid/1
  Switch/1 -> pktBits/1
  Packetized Streams/4(frameStartOut) -> Switch3/1
  Packetized Streams/3(frameEndOut) -> Switch2/1
  Packetized Streams/2(pktValid) -> Switch1/1
  Packetized Streams/1(pktBits) -> Switch/1
  validIn/1 -> Packetized Streams/4(validIn), Continuous Streams/2(validIn)
  endIn/1 -> Packetized Streams/3(endIn)
  startIn/1 -> Packetized Streams/2(startIn)
  dataIn/1 -> Packetized Streams/1(dataIn), Continuous Streams/1(dataIn)

== system dvbs2_stream/HDL_DUT/Tx/DVB-S2 Tx/BB Frame Generator/BB Header and Data CRC Generator/No HDL ==
  In2 : Inport
  u : Inport  Port=2
  vld : Inport  Port=3
  Logical Operator3 : Logic  Operator=NOT  AllPortsSameDT=off  OutDataTypeStr=boolean
  Logical Operator4 : Logic  AllPortsSameDT=off  OutDataTypeStr=boolean
  Logical Operator5 : Logic  Operator=NOT  AllPortsSameDT=off  OutDataTypeStr=boolean
  MATLAB Function1 : MATLAB Function  TreatAsAtomicUnit=on
  No HDL : Subsystem
  wires:
  Logical Operator3/1 -> Logical Operator4/1
  MATLAB Function1/1(y) -> Logical Operator5/1
  u/1 -> MATLAB Function1/1(u)
  vld/1 -> No HDL/2(vld)
  Logical Operator5/1 -> Logical Operator4/2
  Logical Operator4/1 -> No HDL/1(rdy)
  In2/1 -> Logical Operator3/1

== system dvbs2_stream/HDL_DUT/Tx/DVB-S2 Tx/BB Frame Generator/BB Scrambler/Subsystem ==
  In1 : Inport
  Enable : EnablePort
  PN Sequence Generator : commseqgen3/PN Sequence Generator  poly='z^15 + z + 1'  ini_sta=[1 0 0 1 0 1 0 1 0 0 0 0 0 0 0]  outBitMaskSource=Dialog parameter  shift=15  outVarSiz=off  maxOutSizeMode=Dialog parameter  maxOutSize=[10 1]  Ts=-1  sampPerFrame=1  reset=on  bitPackedOutputs=off  outDataType=Smallest unsigned integer  numPackedBits=8  bitPackDataSigned=off  bitPackedOutDType=double
  Out1 : Outport  InitialOutput=0
  wires:
  PN Sequence Generator/1 -> Out1/1
  In1/1 -> PN Sequence Generator/1

== system dvbs2_stream/HDL_DUT/Tx/DVB-S2 Tx/BB Frame Generator/Data Store FIFO/No HDL ==
  rd : Inport
  wr : Inport  Port=2
  No HDL : Subsystem
  RAM status : MATLAB Function  TreatAsAtomicUnit=on
  wires:
  RAM status/2(ncount) -> No HDL/3(ncount)
  RAM status/3(empty) -> No HDL/4(empty)
  RAM status/1(full) -> No HDL/2(full)
  wr/1 -> RAM status/1(wr), No HDL/1(wr)
  rd/1 -> RAM status/2(rd), No HDL/5(rd)

== system dvbs2_stream/HDL_DUT/Tx/DVB-S2 Tx/BB Frame Generator/Multiplexer/No HDL ==
  dvalid : Inport
  hvalid : Inport  Port=2
  Assertion : Assertion
  Delay : Delay  DelayLength=10
  Logical Operator1 : Logic  AllPortsSameDT=off  OutDataTypeStr=boolean
  Logical Operator2 : Logic  Operator=NOT  AllPortsSameDT=off  OutDataTypeStr=boolean
  wires:
  Delay/1 -> Logical Operator2/1
  dvalid/1 -> Logical Operator1/1
  Logical Operator1/1 -> Delay/1
  hvalid/1 -> Logical Operator1/2
  Logical Operator2/1 -> Assertion/1

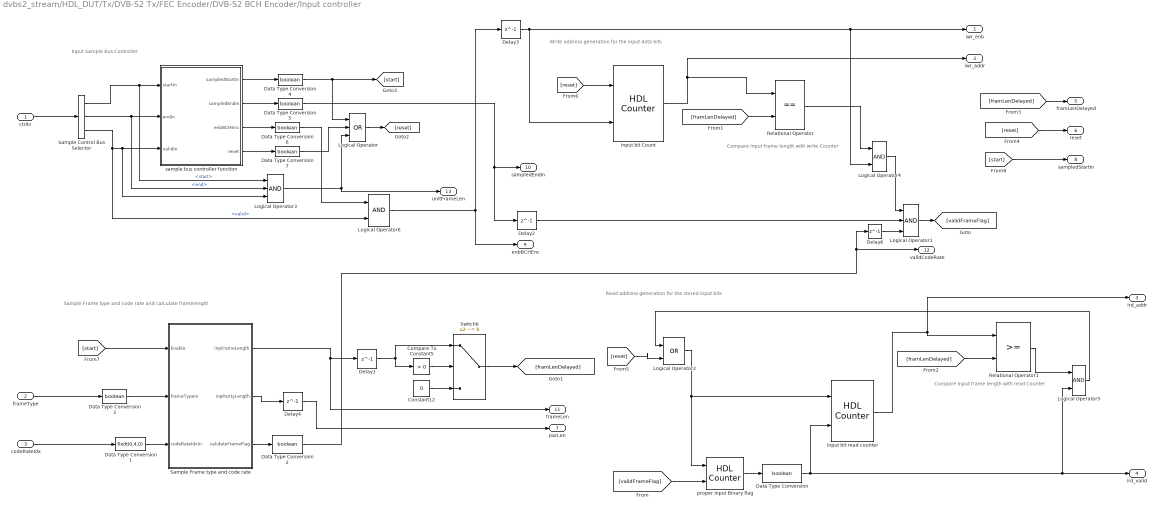
== system dvbs2_stream/HDL_DUT/Tx/DVB-S2 Tx/FEC Encoder/DVB-S2 BCH Encoder/Input controller ==
  note: Input Sample Bus Controller
  note: Compare input frame length with read Counter
  note: Compare input frame length with write Counter
  note: Sample Frame type and code rate and calculate framelength
  note: Write address generation for the input data bits
  note: Read address generation for the stored input bits
  ctrlIn : Inport
  frameType : Inport  Port=2
  codeRateIdx : Inport  Port=3
  Compare To Constant5 : simulink/Logic and Bit Operations/Compare To Constant  relop=>  const=0  OutDataTypeStr=boolean
  Constant12 : Constant  Value=0  OutDataTypeStr=Inherit: Inherit via back propagation  SampleTime=-1
  Data Type Conversion{,2,4..7} (6 alike) : DataTypeConversion  OutDataTypeStr=boolean  SaturateOnIntegerOverflow=off  RndMeth=Floor
  Data Type Conversion1 : DataTypeConversion  OutDataTypeStr=fixdt(0,4,0)  RndMeth=Nearest  SaturateOnIntegerOverflow=off
  Data Type Conversion3 : DataTypeConversion  OutDataTypeStr=boolean  RndMeth=Nearest  SaturateOnIntegerOverflow=off
  Delay{1..4,6} (5 alike) : Delay  DelayLength=1
  Input bit Count : hdlsllib/Sources/HDL Counter  CountType=Count limited  CountInit=0  CountStep=1  CountMax=65535  CountFromType=Initial value  CountFrom=0  CountResetPort=on  CountLoadPort=off  CountEnbPort=on  CountDirPort=off  CountHitOutputPort=off  CountDataType=Unsigned  CountWordLen=16  CountFracLen=0  CountSampTime=1
  Logical Operator : Logic  Operator=OR  Inputs=3  IconShape=distinctive  AllPortsSameDT=off  OutDataTypeStr=boolean
  Logical Operator1 : Logic  Inputs=3  IconShape=distinctive  AllPortsSameDT=off  OutDataTypeStr=boolean
  Logical Operator2 : Logic  Operator=OR  IconShape=distinctive  AllPortsSameDT=off  OutDataTypeStr=boolean
  Logical Operator3 : Logic  Inputs=3  IconShape=distinctive  AllPortsSameDT=off  OutDataTypeStr=boolean
  Logical Operator4 : Logic  IconShape=distinctive  AllPortsSameDT=off  OutDataTypeStr=boolean
  Logical Operator5 : Logic  IconShape=distinctive  AllPortsSameDT=off  OutDataTypeStr=boolean
  Logical Operator6 : Logic  IconShape=distinctive  AllPortsSameDT=off  OutDataTypeStr=boolean
  Relational Operator : RelationalOperator  Operator===  OutDataTypeStr=boolean  InputSameDT=off
  Relational Operator1 : RelationalOperator  OutDataTypeStr=boolean  InputSameDT=off
  Sample Control Bus Selector : whdlutilities/Sample Control Bus Selector  OutputSignals=start,end,valid
  Sample Frame type and code rate : MATLAB Function  TreatAsAtomicUnit=on
  Switch6 : Switch  Criteria=u2 ~= 0  SaturateOnIntegerOverflow=off  InputSameDT=off
  input bit read counter : hdlsllib/Sources/HDL Counter  CountType=Count limited  CountInit=0  CountStep=1  CountMax=65535  CountFromType=Initial value  CountFrom=0  CountResetPort=on  CountLoadPort=off  CountEnbPort=on  CountDirPort=off  CountHitOutputPort=off  CountDataType=Unsigned  CountWordLen=16  CountFracLen=0  CountSampTime=1
  proper Input Binary flag : hdlsllib/Sources/HDL Counter  CountType=Count limited  CountInit=0  CountStep=1  CountMax=1  CountFromType=Initial value  CountFrom=0  CountResetPort=on  CountLoadPort=off  CountEnbPort=on  CountDirPort=off  CountHitOutputPort=off  CountDataType=Unsigned  CountWordLen=1  CountFracLen=0  CountSampTime=1
  sample bus controller function : MATLAB Function  TreatAsAtomicUnit=on
  iwr_enb : Outport
  iwr_addr : Outport  Port=2
  ird_addr : Outport  Port=3
  ird_valid : Outport  Port=4
  framLenDelayed : Outport  Port=5
  reset : Outport  Port=6
  parLen : Outport  Port=7
  sampledStartIn : Outport  Port=8
  enbBCHEnc : Outport  Port=9
  sampledEndIn : Outport  Port=10
  frameLen : Outport  Port=11
  validCodeRate : Outport  Port=12
  unitFrameLen : Outport  Port=13
  wires:
  Input bit Count/1 -> iwr_addr/1, Relational Operator/1
  Data Type Conversion2/1 -> Delay6/1, validCodeRate/1
  input bit read counter/1 -> ird_addr/1, Relational Operator1/1
  Data Type Conversion/1 -> Logical Operator5/2, ird_valid/1, input bit read counter/2
  Sample Frame type and code rate/1(inpFrameLength) -> frameLen/1, Delay1/1
  Delay3/1 -> iwr_enb/1, Logical Operator4/2, Input bit Count/2
  Logical Operator3/1 -> unitFrameLen/1, Logical Operator/3
  Delay4/1 -> parLen/1
  [validFrameFlag] -> proper Input Binary flag/2
  Delay6/1 -> Logical Operator1/3
  Sample Frame type and code rate/3(validateFrameFlag) -> Data Type Conversion2/1
  Relational Operator1/1 -> Logical Operator5/1
  Relational Operator/1 -> Logical Operator4/1
  Sample Frame type and code rate/2(inpParityLength) -> Delay4/1
  Logical Operator5/1 -> Logical Operator2/1
  Logical Operator2/1 -> proper Input Binary flag/1, input bit read counter/1
  proper Input Binary flag/1 -> Data Type Conversion/1
  Logical Operator1/1 -> [validFrameFlag]
  Delay2/1 -> Logical Operator1/2
  Data Type Conversion5/1 -> Delay2/1, sampledEndIn/1
  Delay1/1 -> Compare To Constant5/1, Switch6/1
  Data Type Conversion4/1 -> [start], Logical Operator/1
  Logical Operator6/1 -> enbBCHEnc/1, Delay3/1
  codeRateIdx/1 -> Data Type Conversion1/1
  frameType/1 -> Data Type Conversion3/1
  Data Type Conversion1/1 -> Sample Frame type and code rate/3(codeRateIdxIn)
  Logical Operator4/1 -> Logical Operator1/1
  Data Type Conversion3/1 -> Sample Frame type and code rate/2(frameTypeIn)
  Constant12/1 -> Switch6/3
  Compare To Constant5/1 -> Switch6/2
  Data Type Conversion6/1 -> Logical Operator6/1
  Data Type Conversion7/1 -> Logical Operator/2
  Sample Control Bus Selector/1 -> Logical Operator3/1, sample bus controller function/1(startIn)  "<start>"
  ctrlIn/1 -> Sample Control Bus Selector/1
  Sample Control Bus Selector/3 -> Logical Operator6/2, Logical Operator3/3, sample bus controller function/3(validIn)  "<valid>"
  sample bus controller function/2(sampledEndIn) -> Data Type Conversion5/1
  sample bus controller function/3(enbBCHEnc) -> Data Type Conversion6/1
  Sample Control Bus Selector/2 -> Logical Operator3/2, sample bus controller function/2(endIn)  "<end>"
  sample bus controller function/4(reset) -> Data Type Conversion7/1
  sample bus controller function/1(sampledStartIn) -> Data Type Conversion4/1
  Switch6/1 -> [framLenDelayed]
  [framLenDelayed] -> Relational Operator/2
  [framLenDelayed] -> Relational Operator1/2
  [framLenDelayed] -> framLenDelayed/1
  Logical Operator/1 -> [reset]
  [reset] -> reset/1
  [reset] -> Logical Operator2/2
  [reset] -> Input bit Count/1
  [start] -> Sample Frame type and code rate/1(Enable)
  [start] -> sampledStartIn/1
